simulink model "SEVEN_TAP_FILTER_USING_BLOCKS"  (R2022b)
settings: Solver=FixedStepDiscrete  StartTime=0.0  StopTime=10.0  RelTol=1e-3
libraries: dspsrcs4 x1
settings Model: DataTypeOverride=Off  Creator=saran  LastModifiedBy=saran
settings SolverCC: AlgebraicLoopSolver=TrustRegion
settings DataIOCC: LimitDataPoints=on  SaveOutput=off  SaveTime=off
settings OptimizationCC: BlockReduction=off  ConditionallyExecuteInputs=off  DefaultParameterBehavior=Inlined  DefaultUnderspecifiedDataType=single  LifeSpan=inf
settings DebuggingCC: AlgebraicLoopMsg=error  SingleTaskRateTransMsg=error  UnconnectedInputMsg=warning  UnconnectedOutputMsg=warning  UnconnectedLineMsg=warning  AllowSymbolicDim=off  StrictBusMsg=ErrorOnBusTreatedAsVector  SFUnexpectedBacktrackingDiag=warning  SFNoUnconditionalDefaultTransitionDiag=warning  SFExecutionAtInitializationDiag=none  SFMachineParentedDataDiag=warning  ArithmeticOperatorsInVariantConditions=warning
settings HardwareCC: ProdBitPerPointer=32  ProdBitPerSizeT=32  ProdBitPerPtrDiffT=32  ProdLargestAtomicFloat=None  ProdIntDivRoundTo=Undefined  ProdEndianess=Unspecified  ProdWordSize=32  ProdHWDeviceType=ASIC/FPGA->ASIC/FPGA  ProdEqTarget=off
settings ModelReferenceCC: EnableRefExpFcnMdlSchedulingChecks=on
settings SFSimCC: SimUseLocalCustomCode=off  CustomCodeUndefinedFunction=UseInterfaceOnly
settings RTWCC: RTWUseLocalCustomCode=off
settings CodeAppCC: StateflowObjectComments=on
settings GRTTargetCC: TargetLangStandard=C89/C90 (ANSI)
settings ConfigComp: CovScope=ReferencedModels  CovMetricSettings=dw  CovSaveCumulativeToWorkspaceVar=on  CovSaveSingleToWorkspaceVar=on  CovExternalEMLEnable=off  CovSFcnEnable=off

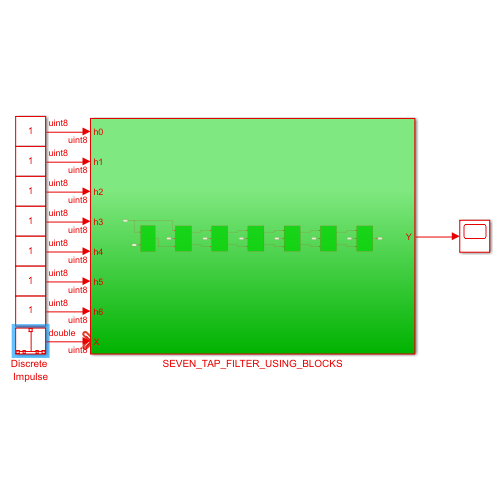
[thumbnail: Simulink's stored preview of the top-level diagram]
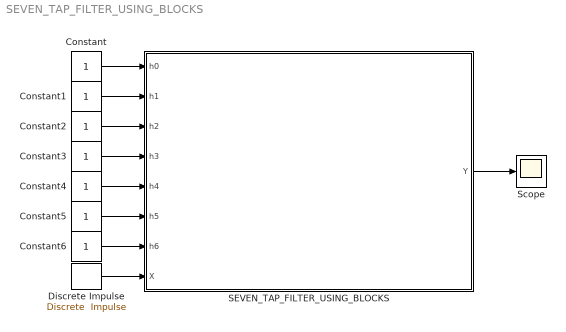
== system SEVEN_TAP_FILTER_USING_BLOCKS ==
  Constant{,1..6} (7 alike) : Constant  OutDataTypeStr=uint8  SampleTime=1
  Discrete Impulse : dspsrcs4/Discrete  Impulse  Delay=0  SampleTime=1  FrameSample=1  OutputFrames=off  dataType=uint8  isSigned=on  wordLen=16  udDataType=sfix(16)  fracBitsMode=Best precision  numFracBits=15  OutDataTypeStr=uint8  LastOutDataTypeStr=uint8
  SEVEN_TAP_FILTER_USING_BLOCKS : Subsystem
  Scope : Scope
  wires:
  SEVEN_TAP_FILTER_USING_BLOCKS/1(Y) -> Scope/1
  Constant/1 -> SEVEN_TAP_FILTER_USING_BLOCKS/1(h0)
  Constant1/1 -> SEVEN_TAP_FILTER_USING_BLOCKS/2(h1)
  Constant2/1 -> SEVEN_TAP_FILTER_USING_BLOCKS/3(h2)
  Constant3/1 -> SEVEN_TAP_FILTER_USING_BLOCKS/4(h3)
  Constant4/1 -> SEVEN_TAP_FILTER_USING_BLOCKS/5(h4)
  Constant5/1 -> SEVEN_TAP_FILTER_USING_BLOCKS/6(h5)
  Constant6/1 -> SEVEN_TAP_FILTER_USING_BLOCKS/7(h6)
  Discrete Impulse/1 -> SEVEN_TAP_FILTER_USING_BLOCKS/8(X)

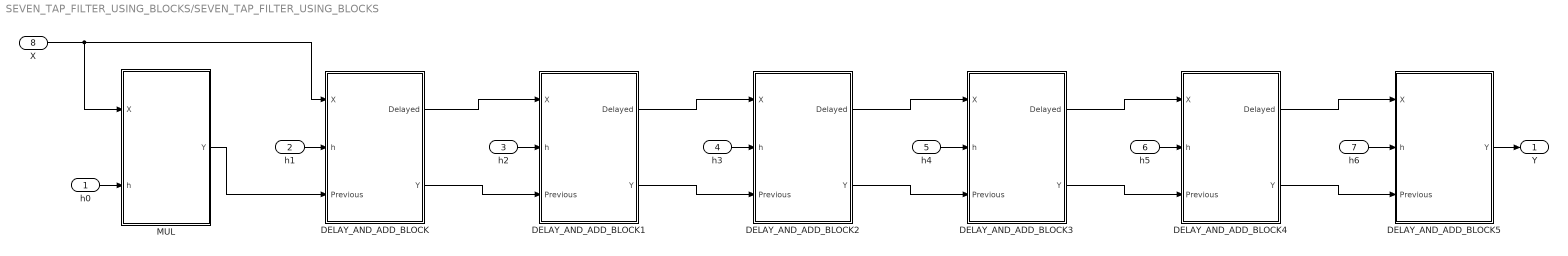
== system SEVEN_TAP_FILTER_USING_BLOCKS/SEVEN_TAP_FILTER_USING_BLOCKS ==
  h0 : Inport  OutDataTypeStr=uint8  SampleTime=1  LockScale=on
  h1 : Inport  Port=2  OutDataTypeStr=uint8  SampleTime=1  LockScale=on
  h2 : Inport  Port=3  OutDataTypeStr=uint8  SampleTime=1  LockScale=on
  h3 : Inport  Port=4  OutDataTypeStr=uint8  SampleTime=1  LockScale=on
  h4 : Inport  Port=5  OutDataTypeStr=uint8  SampleTime=1  LockScale=on
  h5 : Inport  Port=6  OutDataTypeStr=uint8  SampleTime=1  LockScale=on
  h6 : Inport  Port=7  OutDataTypeStr=uint8  SampleTime=1  LockScale=on
  X : Inport  Port=8
  DELAY_AND_ADD_BLOCK : Subsystem
  DELAY_AND_ADD_BLOCK1 : Subsystem
  DELAY_AND_ADD_BLOCK2 : Subsystem
  DELAY_AND_ADD_BLOCK3 : Subsystem
  DELAY_AND_ADD_BLOCK4 : Subsystem
  DELAY_AND_ADD_BLOCK5 : Subsystem
  MUL : Subsystem
  Y : Outport  VectorParamsAs1DForOutWhenUnconnected=off
  wires:
  MUL/1(Y) -> DELAY_AND_ADD_BLOCK/3(Previous)
  h0/1 -> MUL/2(h)
  h1/1 -> DELAY_AND_ADD_BLOCK/2(h)
  h2/1 -> DELAY_AND_ADD_BLOCK1/2(h)
  h3/1 -> DELAY_AND_ADD_BLOCK2/2(h)
  h4/1 -> DELAY_AND_ADD_BLOCK3/2(h)
  h5/1 -> DELAY_AND_ADD_BLOCK4/2(h)
  h6/1 -> DELAY_AND_ADD_BLOCK5/2(h)
  DELAY_AND_ADD_BLOCK/1(Delayed) -> DELAY_AND_ADD_BLOCK1/1(X)
  DELAY_AND_ADD_BLOCK1/1(Delayed) -> DELAY_AND_ADD_BLOCK2/1(X)
  DELAY_AND_ADD_BLOCK2/1(Delayed) -> DELAY_AND_ADD_BLOCK3/1(X)
  DELAY_AND_ADD_BLOCK/2(Y) -> DELAY_AND_ADD_BLOCK1/3(Previous)
  DELAY_AND_ADD_BLOCK1/2(Y) -> DELAY_AND_ADD_BLOCK2/3(Previous)
  DELAY_AND_ADD_BLOCK2/2(Y) -> DELAY_AND_ADD_BLOCK3/3(Previous)
  DELAY_AND_ADD_BLOCK3/1(Delayed) -> DELAY_AND_ADD_BLOCK4/1(X)
  DELAY_AND_ADD_BLOCK3/2(Y) -> DELAY_AND_ADD_BLOCK4/3(Previous)
  DELAY_AND_ADD_BLOCK4/1(Delayed) -> DELAY_AND_ADD_BLOCK5/1(X)
  DELAY_AND_ADD_BLOCK4/2(Y) -> DELAY_AND_ADD_BLOCK5/3(Previous)
  X/1 -> MUL/1(X), DELAY_AND_ADD_BLOCK/1(X)
  DELAY_AND_ADD_BLOCK5/1(Y) -> Y/1

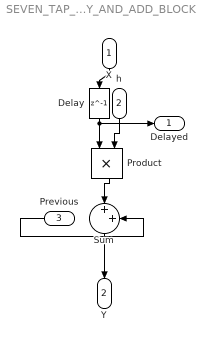
== system SEVEN_TAP_FILTER_USING_BLOCKS/SEVEN_TAP_FILTER_USING_BLOCKS/DELAY_AND_ADD_BLOCK ==
  X : Inport  OutDataTypeStr=uint8  SampleTime=1
  h : Inport  Port=2  OutDataTypeStr=uint8  SampleTime=1
  Previous : Inport  Port=3  OutDataTypeStr=uint8  SampleTime=1
  Delay : Delay  DelayLength=1  InitialCondition=0
  Product : Product
  Sum : Sum  Inputs=|++  AccumDataTypeStr=uint8  OutDataTypeStr=uint8  LockScale=on
  Delayed : Outport  OutDataTypeStr=uint8  SampleTime=1  VectorParamsAs1DForOutWhenUnconnected=off
  Y : Outport  Port=2  OutDataTypeStr=uint8  SampleTime=1  VectorParamsAs1DForOutWhenUnconnected=off
  wires:
  h/1 -> Product/2
  X/1 -> Delay/1
  Delay/1 -> Product/1, Delayed/1
  Product/1 -> Sum/1
  Previous/1 -> Sum/2
  Sum/1 -> Y/1

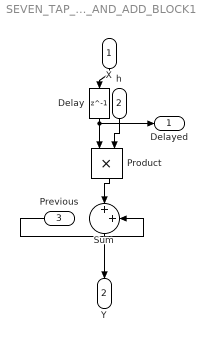
== system SEVEN_TAP_FILTER_USING_BLOCKS/SEVEN_TAP_FILTER_USING_BLOCKS/DELAY_AND_ADD_BLOCK1 ==
  X : Inport  OutDataTypeStr=uint8  SampleTime=1
  h : Inport  Port=2  OutDataTypeStr=uint8  SampleTime=1
  Previous : Inport  Port=3  OutDataTypeStr=uint8  SampleTime=1
  Delay : Delay  DelayLength=1  InitialCondition=0
  Product : Product
  Sum : Sum  Inputs=|++  AccumDataTypeStr=uint8  OutDataTypeStr=uint8  LockScale=on
  Delayed : Outport  OutDataTypeStr=uint8  SampleTime=1  VectorParamsAs1DForOutWhenUnconnected=off
  Y : Outport  Port=2  OutDataTypeStr=uint8  SampleTime=1  VectorParamsAs1DForOutWhenUnconnected=off
  wires:
  h/1 -> Product/2
  X/1 -> Delay/1
  Delay/1 -> Product/1, Delayed/1
  Product/1 -> Sum/1
  Previous/1 -> Sum/2
  Sum/1 -> Y/1

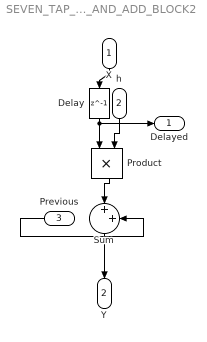
== system SEVEN_TAP_FILTER_USING_BLOCKS/SEVEN_TAP_FILTER_USING_BLOCKS/DELAY_AND_ADD_BLOCK2 ==
  X : Inport  OutDataTypeStr=uint8  SampleTime=1
  h : Inport  Port=2  OutDataTypeStr=uint8  SampleTime=1
  Previous : Inport  Port=3  OutDataTypeStr=uint8  SampleTime=1
  Delay : Delay  DelayLength=1  InitialCondition=0
  Product : Product
  Sum : Sum  Inputs=|++  AccumDataTypeStr=uint8  OutDataTypeStr=uint8  LockScale=on
  Delayed : Outport  OutDataTypeStr=uint8  SampleTime=1  VectorParamsAs1DForOutWhenUnconnected=off
  Y : Outport  Port=2  OutDataTypeStr=uint8  SampleTime=1  VectorParamsAs1DForOutWhenUnconnected=off
  wires:
  h/1 -> Product/2
  X/1 -> Delay/1
  Delay/1 -> Product/1, Delayed/1
  Product/1 -> Sum/1
  Previous/1 -> Sum/2
  Sum/1 -> Y/1

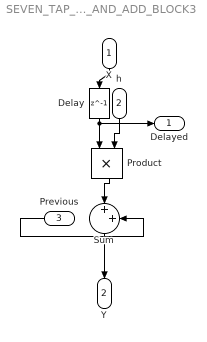
== system SEVEN_TAP_FILTER_USING_BLOCKS/SEVEN_TAP_FILTER_USING_BLOCKS/DELAY_AND_ADD_BLOCK3 ==
  X : Inport  OutDataTypeStr=uint8  SampleTime=1
  h : Inport  Port=2  OutDataTypeStr=uint8  SampleTime=1
  Previous : Inport  Port=3  OutDataTypeStr=uint8  SampleTime=1
  Delay : Delay  DelayLength=1  InitialCondition=0
  Product : Product
  Sum : Sum  Inputs=|++  AccumDataTypeStr=uint8  OutDataTypeStr=uint8  LockScale=on
  Delayed : Outport  OutDataTypeStr=uint8  SampleTime=1  VectorParamsAs1DForOutWhenUnconnected=off
  Y : Outport  Port=2  OutDataTypeStr=uint8  SampleTime=1  VectorParamsAs1DForOutWhenUnconnected=off
  wires:
  h/1 -> Product/2
  X/1 -> Delay/1
  Delay/1 -> Product/1, Delayed/1
  Product/1 -> Sum/1
  Previous/1 -> Sum/2
  Sum/1 -> Y/1

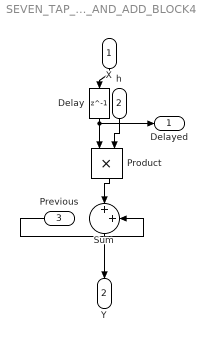
== system SEVEN_TAP_FILTER_USING_BLOCKS/SEVEN_TAP_FILTER_USING_BLOCKS/DELAY_AND_ADD_BLOCK4 ==
  X : Inport  OutDataTypeStr=uint8  SampleTime=1
  h : Inport  Port=2  OutDataTypeStr=uint8  SampleTime=1
  Previous : Inport  Port=3  OutDataTypeStr=uint8  SampleTime=1
  Delay : Delay  DelayLength=1  InitialCondition=0
  Product : Product
  Sum : Sum  Inputs=|++  AccumDataTypeStr=uint8  OutDataTypeStr=uint8  LockScale=on
  Delayed : Outport  OutDataTypeStr=uint8  SampleTime=1  VectorParamsAs1DForOutWhenUnconnected=off
  Y : Outport  Port=2  OutDataTypeStr=uint8  SampleTime=1  VectorParamsAs1DForOutWhenUnconnected=off
  wires:
  h/1 -> Product/2
  X/1 -> Delay/1
  Delay/1 -> Product/1, Delayed/1
  Product/1 -> Sum/1
  Previous/1 -> Sum/2
  Sum/1 -> Y/1

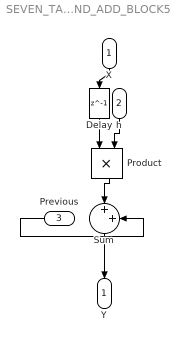
== system SEVEN_TAP_FILTER_USING_BLOCKS/SEVEN_TAP_FILTER_USING_BLOCKS/DELAY_AND_ADD_BLOCK5 ==
  X : Inport  OutDataTypeStr=uint8  SampleTime=1
  h : Inport  Port=2  OutDataTypeStr=uint8  SampleTime=1
  Previous : Inport  Port=3  OutDataTypeStr=uint8  SampleTime=1
  Delay : Delay  DelayLength=1  InitialCondition=0
  Product : Product
  Sum : Sum  Inputs=|++  AccumDataTypeStr=uint8  OutDataTypeStr=uint8  LockScale=on
  Y : Outport  OutDataTypeStr=uint8  SampleTime=1  VectorParamsAs1DForOutWhenUnconnected=off
  wires:
  h/1 -> Product/2
  X/1 -> Delay/1
  Delay/1 -> Product/1
  Product/1 -> Sum/1
  Previous/1 -> Sum/2
  Sum/1 -> Y/1

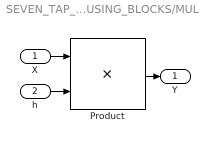
== system SEVEN_TAP_FILTER_USING_BLOCKS/SEVEN_TAP_FILTER_USING_BLOCKS/MUL ==
  X : Inport  OutDataTypeStr=uint8  SampleTime=1
  h : Inport  Port=2  OutDataTypeStr=uint8  SampleTime=1
  Product : Product  OutDataTypeStr=uint8  LockScale=on
  Y : Outport  OutDataTypeStr=uint8  SampleTime=1  VectorParamsAs1DForOutWhenUnconnected=off
  wires:
  X/1 -> Product/1
  Product/1 -> Y/1
  h/1 -> Product/2
